simulink model "model3_2020"  (R2020a)
settings: Solver=VariableStepAuto  StartTime=0.0  StopTime=10.0  RelTol=1e-3
values from neighbouring files (symbols this model uses):
  A = [-3, 2; 1, -2]    [domaci3.m]
  B = [0; 2]    [domaci3.m]
  C = [0, 1]    [domaci3.m]
  K = acker(A, B, p_cl)    [domaci3.m]
  kr = 1 / dcgain(s * G0 / s)    [domaci3.m]
  L = acker(A', C', p_est)'    [domaci3.m]
  R = 5    [domaci3.m]
  x0 = [2; -2]    [domaci3.m]
settings Model: Creator=Nenad  LastModifiedBy=Nenad

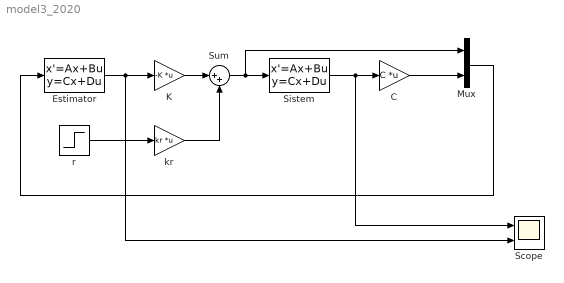
== system model3_2020 ==
  C : Gain  Gain=C  Multiplication=Matrix(K*u) (u vector)
  Estimator : StateSpace  A=A - L * C  B=[B, L]  C=[1, 0; 0, 1]  D=[0, 0; 0, 0]  InitialCondition=[0; 0]
  K : Gain  Gain=-K  Multiplication=Matrix(K*u) (u vector)
  Mux : Mux  Inputs=2
  Scope : Scope  NumInputPorts=2
  Sistem : StateSpace  A=A  B=B  C=[1, 0; 0, 1]  D=[0; 0]  InitialCondition=x0
  Sum : Sum  Inputs=|++
  kr : Gain  Gain=kr  Multiplication=Matrix(K*u) (u vector)
  r : Step  Time=0  After=R  SampleTime=0
  wires:
  Sistem/1 -> Scope/1, C/1
  C/1 -> Mux/2
  Mux/1 -> Estimator/1
  Estimator/1 -> Scope/2, K/1
  Sum/1 -> Mux/1, Sistem/1
  K/1 -> Sum/1
  r/1 -> kr/1
  kr/1 -> Sum/2
